simulink model "Post_Sol_Model_Aug_17"  (R2018a)
settings: Solver=VariableStepAuto  StartTime=0.0  StopTime=1E6  RelTol=1e-3
settings Model: Creator=terry  LastModifiedBy=terry

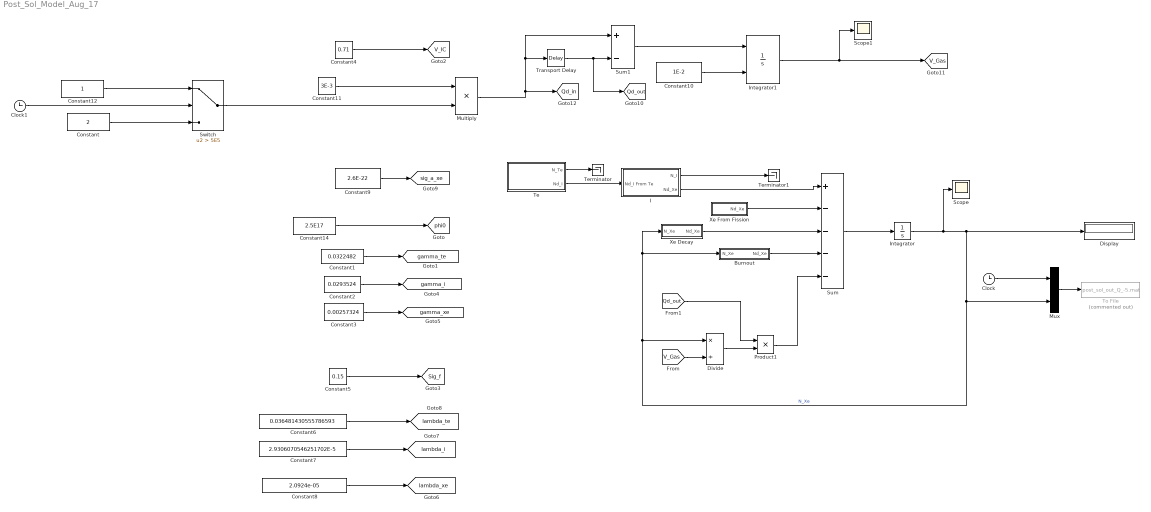
== system Post_Sol_Model_Aug_17 ==
  Burnout : Subsystem
  Clock : Clock
  Clock1 : Clock
  Constant : Constant  Value=2
  Constant1 : Constant  Value=0.0322482
  Constant10 : Constant  Value=1E-2
  Constant11 : Constant  Value=3E-3
  Constant12 : Constant
  Constant14 : Constant  Value=2.5E17
  Constant2 : Constant  Value=0.0293524
  Constant3 : Constant  Value=0.00257324
  Constant4 : Constant  Value=0.71
  Constant5 : Constant  Value=0.15
  Constant6 : Constant  Value=0.036481430555786593
  Constant7 : Constant  Value=2.9306070546251702E-5
  Constant8 : Constant  Value=2.0924e-05
  Constant9 : Constant  Value=2.6E-22
  Display : Display
      settings: Format=short_e
  Divide : Product  Inputs=*/
  I : Subsystem
  Integrator : Integrator  LimitOutput=on  LowerSaturationLimit=0
  Integrator1 : Integrator  InitialConditionSource=external  LimitOutput=on  LowerSaturationLimit=0
  Multiply : Product
  Mux : Mux  Inputs=2
  Product1 : Product
  Scope : Scope
  Scope1 : Scope
  Sum : Sum  Inputs=+----
  Sum1 : Sum  Inputs=+-
  Switch : Switch  Criteria=u2 > Threshold  Threshold=5E5
  Te : Subsystem
  Terminator : Terminator
  Terminator1 : Terminator
  To File : ToFile  Commented=on  Filename=post_sol_out_Q_-5.mat
  Transport Delay : TransportDelay  DelayTime=10
  Xe Decay : Subsystem
  Xe From Fission : Subsystem
  tag scope: Qd_in=global, Qd_out=global, Sig_f=global, V_Gas=global, V_IC=global, gamma_i=global, gamma_te=global, gamma_xe=global, lambda_i=global, lambda_te=global, lambda_xe=global, phi0=global, sig_a_xe=global
  wires:
  Te/1(N_Te) -> Terminator/1
  Te/2(Nd_I) -> I/1(Nd_I From Te)
  I/1(N_I) -> Terminator1/1
  Sum/1 -> Integrator/1
  I/2(Nd_Xe) -> Sum/1
  Xe From Fission/1(Nd_Xe) -> Sum/2
  Xe Decay/1(Nd_Xe) -> Sum/3
  Burnout/1(Nd_Xe) -> Sum/4
  Constant1/1 -> [gamma_te]
  Constant2/1 -> [gamma_i]
  Constant3/1 -> [gamma_xe]
  Constant4/1 -> [V_IC]
  Constant5/1 -> [Sig_f]
  Constant6/1 -> [lambda_te]
  Constant7/1 -> [lambda_i]
  Constant8/1 -> [lambda_xe]
  Constant9/1 -> [sig_a_xe]
  [V_Gas] -> Divide/2
  Divide/1 -> Product1/2
  Product1/1 -> Sum/5
  Constant10/1 -> Integrator1/2
  Integrator1/1 -> Scope1/1, [V_Gas]
  Sum1/1 -> Integrator1/1
  Transport Delay/1 -> [Qd_out], Sum1/2
  [Qd_out] -> Product1/1
  Integrator/1 -> Scope/1, Mux/2, Divide/1, Burnout/1(N_Xe), Xe Decay/1(N_Xe), Display/1  "N_Xe"
  Mux/1 -> To File/1
  Clock/1 -> Mux/1
  Constant14/1 -> [phi0]
  Constant12/1 -> Switch/1
  Clock1/1 -> Switch/2
  Constant/1 -> Switch/3
  Constant11/1 -> Multiply/1
  Multiply/1 -> Transport Delay/1, Sum1/1, [Qd_in]
  Switch/1 -> Multiply/2

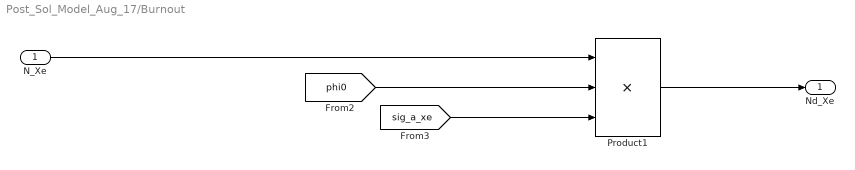
== system Post_Sol_Model_Aug_17/Burnout ==
  N_Xe : Inport
  Product1 : Product  Inputs=3
  Nd_Xe : Outport
  wires:
  N_Xe/1 -> Product1/1
  Product1/1 -> Nd_Xe/1
  [phi0] -> Product1/2
  [sig_a_xe] -> Product1/3

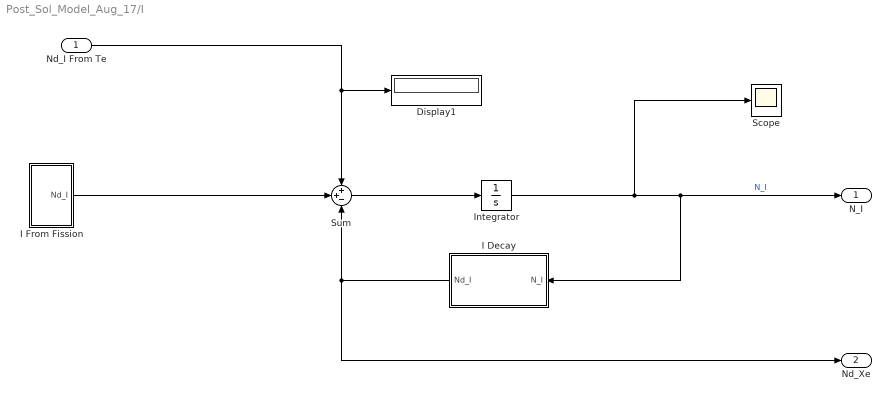
== system Post_Sol_Model_Aug_17/I ==
  Nd_I From Te : Inport
  Display1 : Display
      settings: Format=short_e
  I Decay : Subsystem
  I From Fission : Subsystem
  Integrator : Integrator
  Scope : Scope
  Sum : Sum  Inputs=++-
  N_I : Outport
  Nd_Xe : Outport  Port=2
  wires:
  Integrator/1 -> Scope/1, N_I/1, I Decay/1(N_I)  "N_I"
  Sum/1 -> Integrator/1
  I Decay/1(Nd_I) -> Sum/3, Nd_Xe/1
  Nd_I From Te/1 -> Sum/1, Display1/1
  I From Fission/1(Nd_I) -> Sum/2

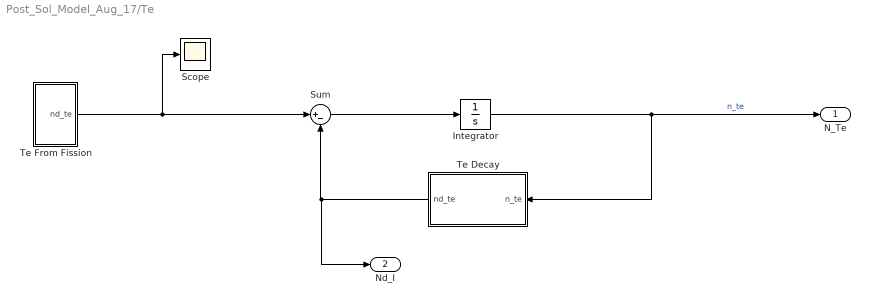
== system Post_Sol_Model_Aug_17/Te ==
  Integrator : Integrator
  Scope : Scope
  Sum : Sum  Inputs=|+-
  Te Decay : Subsystem
  Te From Fission : Subsystem
  N_Te : Outport
  Nd_I : Outport  Port=2
  wires:
  Integrator/1 -> N_Te/1, Te Decay/1(n_te)  "n_te"
  Te Decay/1(nd_te) -> Nd_I/1, Sum/2
  Sum/1 -> Integrator/1
  Te From Fission/1(nd_te) -> Scope/1, Sum/1

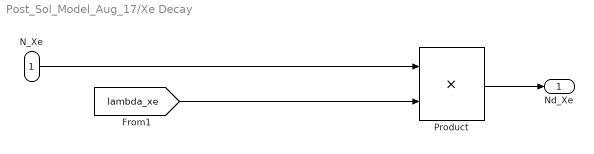
== system Post_Sol_Model_Aug_17/Xe Decay ==
  N_Xe : Inport
  Product : Product
  Nd_Xe : Outport
  wires:
  Product/1 -> Nd_Xe/1
  [lambda_xe] -> Product/2
  N_Xe/1 -> Product/1

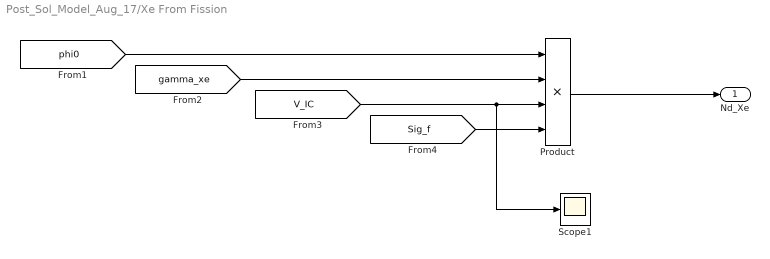
== system Post_Sol_Model_Aug_17/Xe From Fission ==
  Product : Product  Inputs=4
  Scope1 : Scope
  Nd_Xe : Outport
  wires:
  [Sig_f] -> Product/4
  [phi0] -> Product/1
  [gamma_xe] -> Product/2
  [V_IC] -> Scope1/1, Product/3
  Product/1 -> Nd_Xe/1

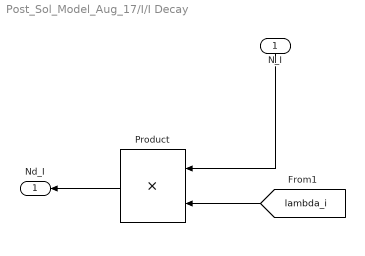
== system Post_Sol_Model_Aug_17/I/I Decay ==
  N_I : Inport
  Product : Product
  Nd_I : Outport
  wires:
  Product/1 -> Nd_I/1
  [lambda_i] -> Product/2
  N_I/1 -> Product/1

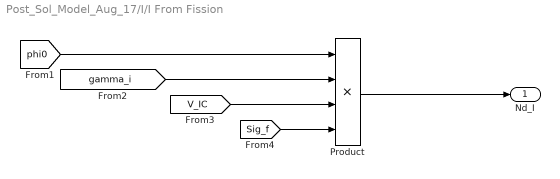
== system Post_Sol_Model_Aug_17/I/I From Fission ==
  Product : Product  Inputs=4
  Nd_I : Outport
  wires:
  [Sig_f] -> Product/4
  [phi0] -> Product/1
  [gamma_i] -> Product/2
  [V_IC] -> Product/3
  Product/1 -> Nd_I/1

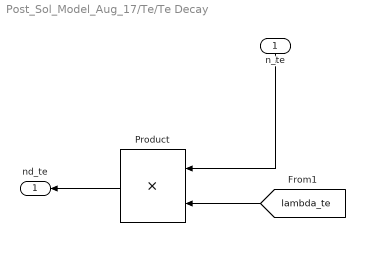
== system Post_Sol_Model_Aug_17/Te/Te Decay ==
  n_te : Inport
  Product : Product
  nd_te : Outport
  wires:
  Product/1 -> nd_te/1
  [lambda_te] -> Product/2
  n_te/1 -> Product/1

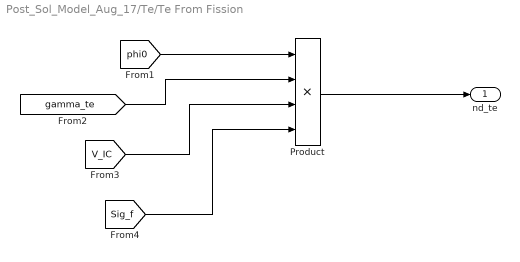
== system Post_Sol_Model_Aug_17/Te/Te From Fission ==
  Product : Product  Inputs=4
  nd_te : Outport
  wires:
  [Sig_f] -> Product/4
  [phi0] -> Product/1
  [gamma_te] -> Product/2
  [V_IC] -> Product/3
  Product/1 -> nd_te/1
